simulink subsystem "GDA_L1AC"  (R2024a)
settings: Solver=VariableStepAuto  StartTime=0.0  StopTime=10.0  RelTol=1e-3
undefined symbols (not defined in the file): Mix
settings Model: Creator=gurt1  LastModifiedBy=gurt1

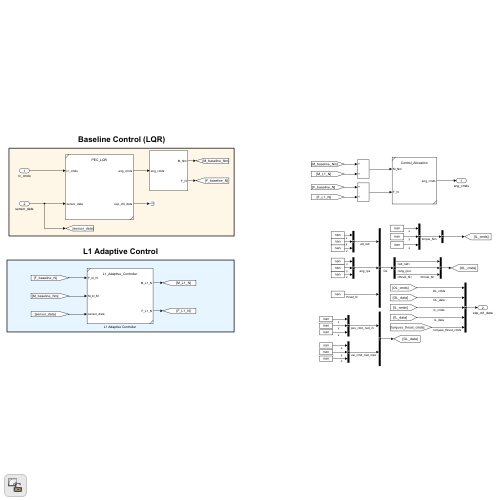
[thumbnail: Simulink's stored preview of the top-level diagram]
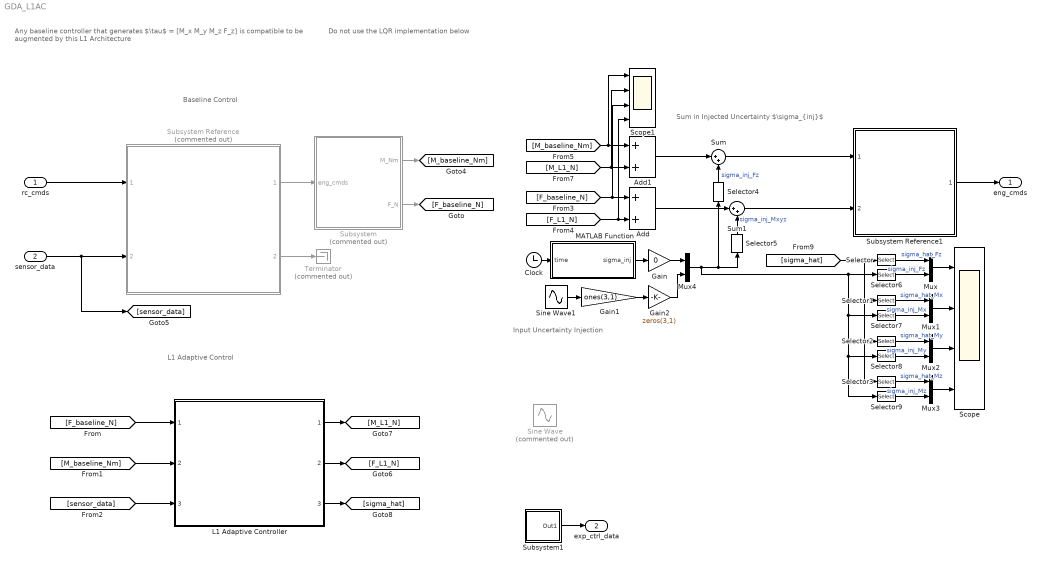
== system GDA_L1AC ==
  note: Any baseline controller that generates $\tau$ = [M_x M_y M_z F_z] is compatible to be augmented by this L1 Architecture
  note: Sum in Injected Uncertainty $\sigma_{inj}$
  note: Baseline Control
  note: L1 Adaptive Control
  note: Input Uncertainty Injection
  note: Do not use the LQR implementation below
  rc_cmds : Inport
  sensor_data : Inport  Port=2
  Add : Sum
  Add1 : Sum
  Clock : Clock
  Gain : Gain  Gain=0
  Gain1 : Gain  Gain=ones(3,1)
  Gain2 : Gain  Gain=zeros(3,1)
  L1 Adaptive Controller : Subsystem  ReferencedSubsystem=L1_Adaptive_Controller
  MATLAB Function : MATLAB Function  TreatAsAtomicUnit=on
  Mux{,1..4} (5 alike) : Mux  Inputs=2
  Scope : Scope  NumInputPorts=4
  Scope1 : Scope  NumInputPorts=4
  Selector : Selector  InputPortWidth=4  IndexOptions=Index vector (dialog)  Indices=1  OutputSizes=1
  Selector1 : Selector  InputPortWidth=4  IndexOptions=Index vector (dialog)  Indices=2  OutputSizes=1
  Selector2 : Selector  InputPortWidth=4  IndexOptions=Index vector (dialog)  Indices=3  OutputSizes=1
  Selector3 : Selector  InputPortWidth=4  IndexOptions=Index vector (dialog)  Indices=4  OutputSizes=1
  Selector4 : Selector  InputPortWidth=4  IndexOptions=Index vector (dialog)  Indices=[2:4]  OutputSizes=1
  Selector5 : Selector  InputPortWidth=4  IndexOptions=Index vector (dialog)  Indices=1  OutputSizes=1
  Selector6 : Selector  InputPortWidth=4  IndexOptions=Index vector (dialog)  Indices=1  OutputSizes=1
  Selector7 : Selector  InputPortWidth=4  IndexOptions=Index vector (dialog)  Indices=2  OutputSizes=1
  Selector8 : Selector  InputPortWidth=4  IndexOptions=Index vector (dialog)  Indices=3  OutputSizes=1
  Selector9 : Selector  InputPortWidth=4  IndexOptions=Index vector (dialog)  Indices=4  OutputSizes=1
  Sine Wave : Sin  Commented=on  Frequency=.5  SampleTime=0
  Sine Wave1 : Sin  Amplitude=2e-3  Frequency=.2  SampleTime=0
  Subsystem : Subsystem  Commented=on
  Subsystem Reference : Subsystem  Commented=on  ReferencedSubsystem=PEC_LQR
  Subsystem Reference1 : Subsystem  ReferencedSubsystem=Control_Allocation
  Subsystem1 : Subsystem
  Sum : Sum  Inputs=|++
  Sum1 : Sum  Inputs=|++
  Terminator : Terminator  Commented=on
  eng_cmds : Outport
  exp_ctrl_data : Outport  Port=2
  wires:
  sensor_data/1 -> Subsystem Reference/2, [sensor_data]
  rc_cmds/1 -> Subsystem Reference/1
  Subsystem Reference/2 -> Terminator/1
  Subsystem Reference/1 -> Subsystem/1(eng_cmds)
  Subsystem/2(F_N) -> [F_baseline_N]
  Subsystem/1(M_Nm) -> [M_baseline_Nm]
  [F_baseline_N] -> L1 Adaptive Controller/1
  [M_baseline_Nm] -> L1 Adaptive Controller/2
  [sensor_data] -> L1 Adaptive Controller/3
  L1 Adaptive Controller/2 -> [F_L1_N]
  L1 Adaptive Controller/1 -> [M_L1_N]
  [F_baseline_N] -> Add/1, Scope1/3
  [F_L1_N] -> Add/2, Scope1/4
  [M_baseline_Nm] -> Add1/1, Scope1/1
  [M_L1_N] -> Add1/2, Scope1/2
  Subsystem Reference1/1 -> eng_cmds/1
  Add1/1 -> Sum/1
  Sum/1 -> Subsystem Reference1/1
  Add/1 -> Sum1/1
  Sum1/1 -> Subsystem Reference1/2
  Clock/1 -> MATLAB Function/1(time)
  MATLAB Function/1(sigma_inj) -> Gain/1
  L1 Adaptive Controller/3 -> [sigma_hat]
  Subsystem1/1(Out1) -> exp_ctrl_data/1
  Mux/1 -> Scope/1
  [sigma_hat] -> Selector/1, Selector1/1, Selector2/1, Selector3/1
  Mux1/1 -> Scope/2
  Mux2/1 -> Scope/3
  Mux3/1 -> Scope/4
  Selector/1 -> Mux/1  "sigma_hat_Fz"
  Selector1/1 -> Mux1/1  "sigma_hat_Mx"
  Selector2/1 -> Mux2/1  "sigma_hat_My"
  Selector3/1 -> Mux3/1  "sigma_hat_Mz"
  Mux4/1 -> Selector5/1, Selector4/1, Selector6/1, Selector7/1, Selector8/1, Selector9/1
  Selector4/1 -> Sum/2  "sigma_inj_Fz"
  Selector5/1 -> Sum1/2  "sigma_inj_Mxyz"
  Selector6/1 -> Mux/2  "sigma_inj_Fz"
  Selector7/1 -> Mux1/2  "sigma_inj_Mx"
  Selector8/1 -> Mux2/2  "sigma_inj_My"
  Selector9/1 -> Mux3/2  "sigma_inj_Mz"
  Gain/1 -> Mux4/1
  Gain1/1 -> Gain2/1
  Gain2/1 -> Mux4/2
  Sine Wave1/1 -> Gain1/1

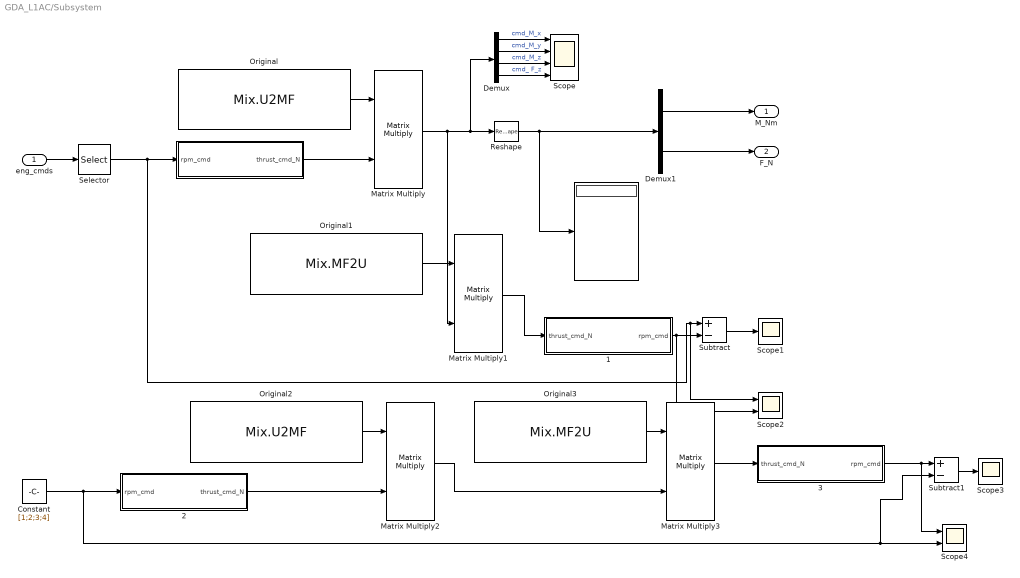
== system GDA_L1AC/Subsystem ==
  eng_cmds : Inport
  "   " : MATLAB Function  TreatAsAtomicUnit=on
  "    " : Display
  "   1" : MATLAB Function  TreatAsAtomicUnit=on
  "   2" : MATLAB Function  TreatAsAtomicUnit=on
  "   3" : MATLAB Function  TreatAsAtomicUnit=on
  " Original" : Constant  Value=Mix.U2MF  OutDataTypeStr=Inherit: Inherit via back propagation  SampleTime=-1
  " Original1" : Constant  Value=Mix.MF2U  OutDataTypeStr=Inherit: Inherit via back propagation  SampleTime=-1
  " Original2" : Constant  Value=Mix.U2MF  OutDataTypeStr=Inherit: Inherit via back propagation  SampleTime=-1
  " Original3" : Constant  Value=Mix.MF2U  OutDataTypeStr=Inherit: Inherit via back propagation  SampleTime=-1
  Constant : Constant  Value=[1;2;3;4]
  Demux : Demux
  Demux1 : Demux  Outputs=[3 1]
  Matrix Multiply{,1..3} (4 alike) : Product  Multiplication=Matrix(*)
  Reshape : Reshape
  Scope : Scope  NumInputPorts=4
  Scope1 : Scope
  Scope2 : Scope  NumInputPorts=2
  Scope3 : Scope
  Scope4 : Scope  NumInputPorts=2
  Selector : Selector  InputPortWidth=16  IndexOptions=Index vector (dialog)  Indices=[1:4]  OutputSizes=1
  Subtract : Sum  Inputs=+-
  Subtract1 : Sum  Inputs=+-
  M_Nm : Outport
  F_N : Outport  Port=2
  wires:
  "   3"/1(rpm_cmd) -> Subtract1/1, Scope4/1
  "   2"/1(thrust_cmd_N) -> Matrix Multiply2/2
  Subtract1/1 -> Scope3/1
  Matrix Multiply3/1 -> "   3"/1(thrust_cmd_N)
  Matrix Multiply2/1 -> Matrix Multiply3/2
  " Original3"/1 -> Matrix Multiply3/1
  Constant/1 -> "   2"/1(rpm_cmd), Scope4/2, Subtract1/2
  " Original2"/1 -> Matrix Multiply2/1
  "   1"/1(rpm_cmd) -> Subtract/2, Scope2/2
  Subtract/1 -> Scope1/1
  Matrix Multiply1/1 -> "   1"/1(thrust_cmd_N)
  "   "/1(thrust_cmd_N) -> Matrix Multiply/2
  " Original1"/1 -> Matrix Multiply1/1
  Demux1/2 -> F_N/1
  Demux1/1 -> M_Nm/1
  Reshape/1 -> "    "/1, Demux1/1
  Demux/2 -> Scope/2  "cmd_M_y"
  Demux/1 -> Scope/1  "cmd_M_x"
  eng_cmds/1 -> Selector/1
  Selector/1 -> "   "/1(rpm_cmd), Subtract/1, Scope2/1
  Matrix Multiply/1 -> Demux/1, Reshape/1, Matrix Multiply1/2
  Demux/4 -> Scope/4  "cmd_ F_z"
  " Original"/1 -> Matrix Multiply/1
  Demux/3 -> Scope/3  "cmd_M_z"

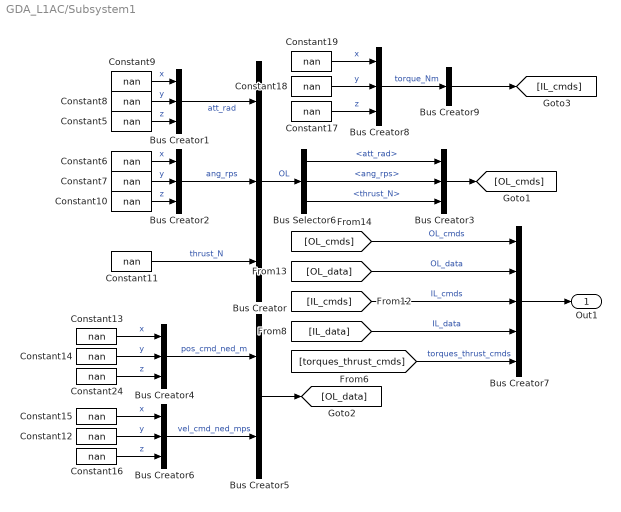
== system GDA_L1AC/Subsystem1 ==
  Bus Creator{,1..4,6,8} (7 alike) : BusCreator  Inputs=3
  Bus Creator5 : BusCreator  Inputs=2
  Bus Creator7 : BusCreator  Inputs=5
  Bus Creator9 : BusCreator  Inputs=1
  Bus Selector6 : BusSelector  OutputSignals=att_rad,ang_rps,thrust_N
  Constant{5..19,24} (16 alike) : Constant  Value=nan
  Out1 : Outport
  wires:
  Bus Creator8/1 -> Bus Creator9/1  "torque_Nm"
  Constant12/1 -> Bus Creator6/2  "y"
  Constant17/1 -> Bus Creator8/3  "z"
  Constant5/1 -> Bus Creator1/3  "z"
  Constant24/1 -> Bus Creator4/3  "z"
  [IL_data] -> Bus Creator7/4  "IL_data"
  Constant6/1 -> Bus Creator2/1  "x"
  Bus Creator7/1 -> Out1/1
  Bus Creator3/1 -> [OL_cmds]
  Constant7/1 -> Bus Creator2/2  "y"
  Constant9/1 -> Bus Creator1/1  "x"
  Constant13/1 -> Bus Creator4/1  "x"
  Bus Selector6/3 -> Bus Creator3/3  "<thrust_N>"
  Constant18/1 -> Bus Creator8/2  "y"
  Bus Creator/1 -> Bus Selector6/1  "OL"
  Bus Selector6/2 -> Bus Creator3/2  "<ang_rps>"
  [IL_cmds] -> Bus Creator7/3  "IL_cmds"
  [torques_thrust_cmds] -> Bus Creator7/5  "torques_thrust_cmds"
  Constant19/1 -> Bus Creator8/1  "x"
  Constant11/1 -> Bus Creator/3  "thrust_N"
  Constant15/1 -> Bus Creator6/1  "x"
  Bus Creator6/1 -> Bus Creator5/2  "vel_cmd_ned_mps"
  Bus Creator2/1 -> Bus Creator/2  "ang_rps"
  [OL_cmds] -> Bus Creator7/1  "OL_cmds"
  Constant16/1 -> Bus Creator6/3  "z"
  Bus Creator5/1 -> [OL_data]
  Constant10/1 -> Bus Creator2/3  "z"
  Bus Creator9/1 -> [IL_cmds]
  [OL_data] -> Bus Creator7/2  "OL_data"
  Constant8/1 -> Bus Creator1/2  "y"
  Bus Selector6/1 -> Bus Creator3/1  "<att_rad>"
  Constant14/1 -> Bus Creator4/2  "y"
  Bus Creator4/1 -> Bus Creator5/1  "pos_cmd_ned_m"
  Bus Creator1/1 -> Bus Creator/1  "att_rad"

== matlab function GDA_L1AC/Subsystem/    ==
  data: rpm_cmd input; thrust_cmd_N output
function thrust_cmd_N = rpm_to_thrust(rpm_cmd)
% Where thrust is in [N]
thrust_cmd_N = (2.09708e-23).*(rpm_cmd.^6) + (-5.45325e-19).*(rpm_cmd.^5) + (4.92327e-15).*(rpm_cmd.^4) + (-1.61462e-11).*(rpm_cmd.^3) ...
          + (1.02953e-7).*(rpm_cmd.^2) + (-1.52264e-5).*rpm_cmd + -1.38011e-2;

== matlab function GDA_L1AC/Subsystem/   1 ==
  data: thrust_cmd_N input; rpm_cmd output
function rpm_cmd = thrust_to_rpm(thrust_cmd_N)
% Where thrust is in [N]
%rpm_cmd = -3.3169.*(thrust_cmd_N.^6) + 67.651.*(thrust_cmd_N.^5) - 532.66.*(thrust_cmd_N.^4) + 2057.2.*(thrust_cmd_N.^3) ...
          %- 4192.7.*(thrust_cmd_N.^2) + 5521.9.*thrust_cmd_N + 623.46;

rpm_cmd = -8.0315127E-02 .* thrust_cmd_N.^6 + ...
           3.1949614E+00 .* thrust_cmd_N.^5 - ...
           4.9699249E+01 .* thrust_cmd_N.^4 + ...
           3.8323911E+02 .* thrust_cmd_N.^3 - ...
           1.5607669E+03 .* thrust_cmd_N.^2 + ...
           4.0014414E+03 .* thrust_cmd_N + ...
           7.6702051E+02;

== matlab function GDA_L1AC/Subsystem/   2 ==
  data: rpm_cmd input; thrust_cmd_N output
function thrust_cmd_N = rpm_to_thrust(rpm_cmd)
% Where thrust is in [N]
% thrust_cmd_N = (2.09708e-23).*(rpm_cmd.^6) + (-5.45325e-19).*(rpm_cmd.^5) + (4.92327e-15).*(rpm_cmd.^4) + (-1.61462e-11).*(rpm_cmd.^3) ...
%           + (1.02953e-7).*(rpm_cmd.^2) + (-1.52264e-5).*rpm_cmd + -1.38011e-2;

thrust_cmd_N = -5.51965E-23 .* rpm_cmd.^6 + ...
               2.19591E-18 .* rpm_cmd.^5 + ...
               -3.31553E-14 .* rpm_cmd.^4 + ...
               2.38718E-10 .* rpm_cmd.^3 + ...
               -7.28773E-07 .* rpm_cmd.^2 + ...
               1.14689E-03 .* rpm_cmd.^1 + ...
               -4.72839E-01;

if thrust_cmd_N < 0
    thrust_cmd_N = 0;
end

== matlab function GDA_L1AC/Subsystem/   3 ==
  data: thrust_cmd_N input; rpm_cmd output
function rpm_cmd = thrust_to_rpm(thrust_cmd_N)
% Where thrust is in [N]
%rpm_cmd = -3.3169.*(thrust_cmd_N.^6) + 67.651.*(thrust_cmd_N.^5) - 532.66.*(thrust_cmd_N.^4) + 2057.2.*(thrust_cmd_N.^3) ...
          %- 4192.7.*(thrust_cmd_N.^2) + 5521.9.*thrust_cmd_N + 623.46;

% rpm_cmd = -8.0315127E-02 .* thrust_cmd_N.^6 + ...
%            3.1949614E+00 .* thrust_cmd_N.^5 - ...
%            4.9699249E+01 .* thrust_cmd_N.^4 + ...
%            3.8323911E+02 .* thrust_cmd_N.^3 - ...
%            1.5607669E+03 .* thrust_cmd_N.^2 + ...
%            4.0014414E+03 .* thrust_cmd_N + ...
%            7.6702051E+02;

rpm_cmd = -1.1387455E-01 .* thrust_cmd_N.^6 + ...
           4.4501328E+00 .* thrust_cmd_N.^5 - ...
           6.7644554E+01 .* thrust_cmd_N.^4 + ...
           5.0554098E+02 .* thrust_cmd_N.^3 - ...
           1.9626185E+03 .* thrust_cmd_N.^2 + ...
           4.5611622E+03 .* thrust_cmd_N + ...
           5.4664025E+02;

if rpm_cmd < 0
    rpm_cmd = 0;
end

== matlab function GDA_L1AC/MATLAB Function ==
  data: time input; sigma_inj output
function sigma_inj = uncertainty(time)

sigma_inj = 0.2*sin(time-20)+0.01*(time-20)+0.15*sin(1.5*(time-20));
